simulink model "sim_complete"  (R2015a)
settings: Solver=ode45  StartTime=0.0  StopTime=10.0  RelTol=1e-3
values from neighbouring files (symbols this model uses):
  params = catstruct(params, sys.params_str)    [double_lqg.m]    (also in load_mechanism_params.m = params(1:13); load_params.m = [g, m0, b0,                m1, I1, b1, L1, L1_cg,           ; load_single_mechanism_params.m = params(1:8); load_single_params.m = [g, m0, b0,                m1, I1, b1, L1, L1_cg,           )
libraries: aerolibutil x1
settings Model: Creator=BPeixoto  LastModifiedBy=BPeixoto

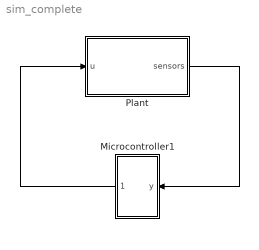
== system sim_complete ==
  Microcontroller1 : Subsystem
  Plant : Subsystem
  wires:
  Microcontroller1/1(PWM) -> Plant/1(u)
  Plant/1(sensors) -> Microcontroller1/1(y)

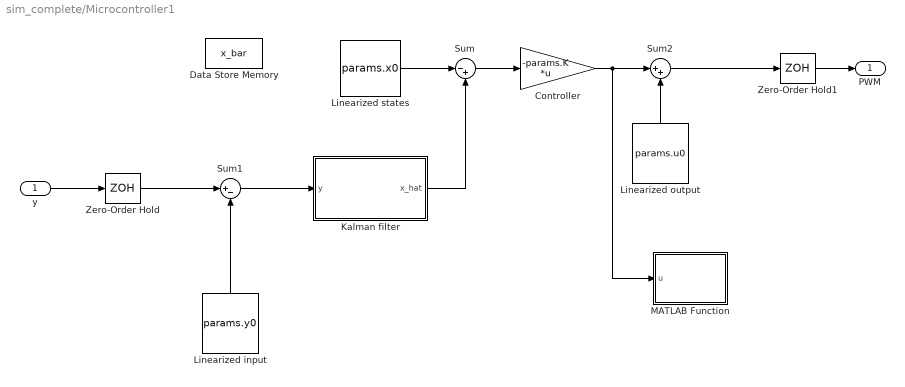
== system sim_complete/Microcontroller1 ==
  y : Inport
  Controller : Gain  Gain=-params.K  Multiplication=Matrix(K*u)
  Data Store Memory : DataStoreMemory  DataStoreName=x_bar  ReadBeforeWriteMsg=warning  WriteAfterWriteMsg=warning  WriteAfterReadMsg=warning  InitialValue=zeros(6, 1)  OutDataTypeStr=double
  Kalman filter : MATLAB Function  TreatAsAtomicUnit=on
  Linearized input : Constant  Value=params.y0
  Linearized output : Constant  Value=params.u0
  Linearized states : Constant  Value=params.x0
  MATLAB Function : MATLAB Function  TreatAsAtomicUnit=on
  Sum : Sum  Inputs=|-+
  Sum1 : Sum  Inputs=|+-
  Sum2 : Sum  Inputs=|++
  Zero-Order Hold : ZeroOrderHold  SampleTime=params.ts
  Zero-Order Hold1 : ZeroOrderHold  SampleTime=params.ts
  PWM : Outport
  wires:
  y/1 -> Zero-Order Hold/1
  Linearized states/1 -> Sum/1
  Sum/1 -> Controller/1
  Linearized input/1 -> Sum1/2
  Zero-Order Hold/1 -> Sum1/1
  Controller/1 -> MATLAB Function/1(u), Sum2/1
  Linearized output/1 -> Sum2/2
  Sum1/1 -> Kalman filter/1(y)
  Sum2/1 -> Zero-Order Hold1/1
  Zero-Order Hold1/1 -> PWM/1
  Kalman filter/1(x_hat) -> Sum/2

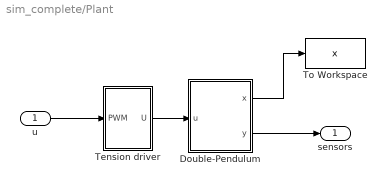
== system sim_complete/Plant ==
  u : Inport
  Double-Pendulum : Subsystem
  Tension driver : Subsystem
  To Workspace : ToWorkspace  VariableName=x  SaveFormat=Timeseries  SampleTime=-1
  sensors : Outport
  wires:
  Double-Pendulum/2(y) -> sensors/1
  Double-Pendulum/1(x) -> To Workspace/1
  u/1 -> Tension driver/1(PWM)
  Tension driver/1(U) -> Double-Pendulum/1(u)

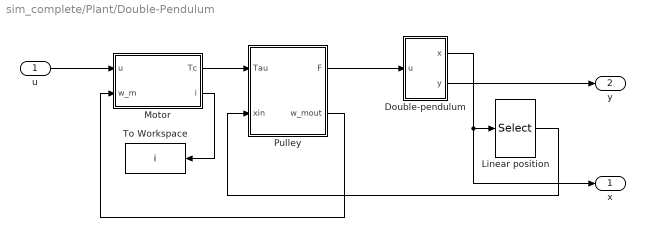
== system sim_complete/Plant/Double-Pendulum ==
  u : Inport
  Double-pendulum : Subsystem
  Linear position : Selector  InputPortWidth=6  Indices=[1]
  Motor : MATLAB Function  TreatAsAtomicUnit=on
  Pulley : Subsystem
  To Workspace : ToWorkspace  VariableName=i  SaveFormat=Timeseries  SampleTime=-1
  x : Outport
  y : Outport  Port=2
  wires:
  u/1 -> Motor/1(u)
  Double-pendulum/1(x) -> x/1, Linear position/1
  Motor/2(i) -> To Workspace/1
  Double-pendulum/2(y) -> y/1
  Motor/1(Tc) -> Pulley/1(Tau)
  Linear position/1 -> Pulley/2(xin)
  Pulley/2(w_mout) -> Motor/2(w_m)
  Pulley/1(F) -> Double-pendulum/1(u)

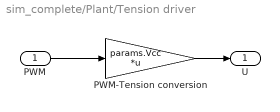
== system sim_complete/Plant/Tension driver ==
  PWM : Inport
  PWM-Tension conversion : Gain  Gain=params.Vcc  Multiplication=Matrix(K*u)
  U : Outport
  wires:
  PWM/1 -> PWM-Tension conversion/1
  PWM-Tension conversion/1 -> U/1

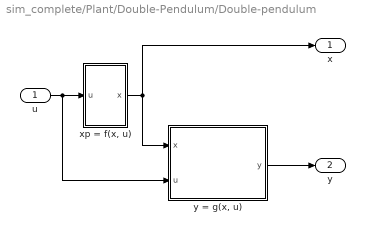
== system sim_complete/Plant/Double-Pendulum/Double-pendulum ==
  u : Inport
  "xp = f(x, u)" : Subsystem
  "y = g(x, u)" : MATLAB Function  TreatAsAtomicUnit=on
  x : Outport
  y : Outport  Port=2
  wires:
  u/1 -> "y = g(x, u)"/2(u), "xp = f(x, u)"/1(u)
  "y = g(x, u)"/1(y) -> y/1
  "xp = f(x, u)"/1(x) -> x/1, "y = g(x, u)"/1(x)

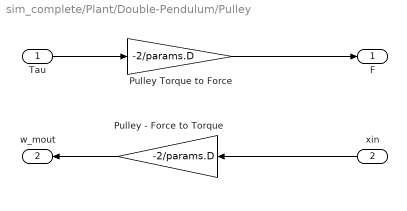
== system sim_complete/Plant/Double-Pendulum/Pulley ==
  Tau : Inport
  xin : Inport  Port=2
  Pulley Torque to Force : Gain  Gain=-2/params.D
  Pulley - Force to Torque : Gain  Gain=-2/params.D
  F : Outport
  w_mout : Outport  Port=2
  wires:
  Pulley Torque to Force/1 -> F/1
  Tau/1 -> Pulley Torque to Force/1
  xin/1 -> Pulley - Force to Torque/1
  Pulley - Force to Torque/1 -> w_mout/1

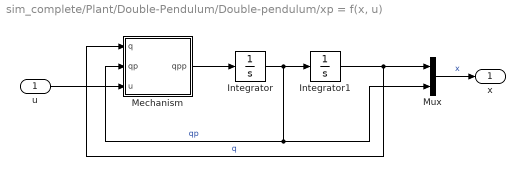
== system sim_complete/Plant/Double-Pendulum/Double-pendulum/xp = f(x, u) ==
  u : Inport
  Integrator : Integrator  InitialCondition=params.qp0
  Integrator1 : Integrator  InitialCondition=params.q0
  Mechanism : Subsystem
  Mux : Mux  Inputs=2
  x : Outport
  wires:
  Mux/1 -> x/1  "x"
  u/1 -> Mechanism/3(u)
  Integrator/1 -> Integrator1/1, Mechanism/2(qp), Mux/2  "qp"
  Mechanism/1(qpp) -> Integrator/1
  Integrator1/1 -> Mux/1, Mechanism/1(q)  "q"

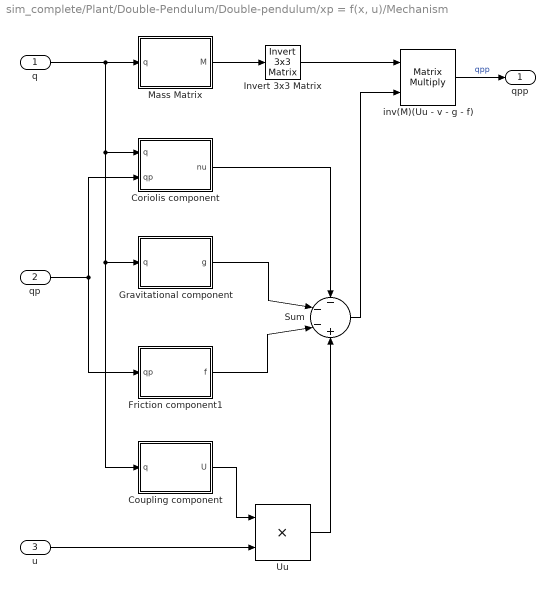
== system sim_complete/Plant/Double-Pendulum/Double-pendulum/xp = f(x, u)/Mechanism ==
  q : Inport
  qp : Inport  Port=2
  u : Inport  Port=3
  Coriolis component : MATLAB Function  TreatAsAtomicUnit=on
  Coupling component : MATLAB Function  TreatAsAtomicUnit=on
  Friction component1 : MATLAB Function  TreatAsAtomicUnit=on
  Gravitational component : MATLAB Function  TreatAsAtomicUnit=on
  Invert 3x3 Matrix : aerolibutil/Invert  3x3 Matrix
  Mass Matrix : MATLAB Function  TreatAsAtomicUnit=on
  Sum : Sum  Inputs=-|-|-|+
  Uu : Product  RndMeth=Nearest
  inv(M)(Uu - v - g - f) : Product  Multiplication=Matrix(*)  OutDataTypeStr=Inherit: Inherit via back propagation  SaturateOnIntegerOverflow=on  InputSameDT=on
  qpp : Outport
  wires:
  Mass Matrix/1(M) -> Invert 3x3 Matrix/1
  Coriolis component/1(nu) -> Sum/1
  qp/1 -> Coriolis component/2(qp), Friction component1/1(qp)
  q/1 -> Coupling component/1(q), Gravitational component/1(q), Coriolis component/1(q), Mass Matrix/1(q)
  Gravitational component/1(g) -> Sum/2
  Friction component1/1(f) -> Sum/3
  Invert 3x3 Matrix/1 -> inv(M)(Uu - v - g - f)/1
  Sum/1 -> inv(M)(Uu - v - g - f)/2
  inv(M)(Uu - v - g - f)/1 -> qpp/1  "qpp"
  Coupling component/1(U) -> Uu/1
  u/1 -> Uu/2
  Uu/1 -> Sum/4

== matlab function sim_complete/Plant/Double-Pendulum/Double-pendulum/xp = f(x, u)/Mechanism/Coriolis component ==
  settings: updateMethod=DISCRETE  sampleTime=params.ts
  data: q input; qp input; nu output; params parameter
function nu = corvec(q, qp, params)
    % Coriolis 'vector
    nu = zeros(3, 1);
    
    % Coupled mass matrix
    nu(1) = -params.m2*params.L2_cg*sin(q(2) + q(3))*(qp(2) + qp(3)^2 ...
            -(params.m2*params.L1 + params.m1*params.L1_cg)*sin(q(2))*qp(3)^2);
    nu(2) = -params.m2*qp(3)*(2*qp(2) + qp(3))*params.L2_cg*params.L1*sin(q(3));
    nu(3) = params.m2*(qp(2)^2)*params.L2_cg*params.L1*sin(q(3));
end

== matlab function sim_complete/Plant/Double-Pendulum/Double-pendulum/xp = f(x, u)/Mechanism/Coupling component ==
  settings: updateMethod=DISCRETE  sampleTime=params.ts
  data: q input; U output
function U = Uvec(q)
    U = [1; 0; 0];
end

== matlab function sim_complete/Microcontroller1/Kalman filter ==
  data: y input; params parameter; u_ant data_store_memory; x_hat_ant data_store_memory; x_hat output
function x_hat = kalman_filter(y, params)
    % First assignemnt
    global x_bar;
    
    % Main matrices
    L = params.L;
    Phi = params.Phi;
    Gamma = params.Gamma;
    C = params.C;
    
    % Time and measurement update
    x_hat = x_bar + L*(y - C*x_bar);
    x_bar = Phi*x_hat + Gamma*u_ant;
end

== matlab function sim_complete/Microcontroller1/MATLAB Function ==
  data: u input; u_ant data_store_memory
function save_uant(u)    
    global u_ant;    
    u_ant = u;
end

== matlab function sim_complete/Plant/Double-Pendulum/Motor ==
  settings: updateMethod=DISCRETE  sampleTime=params.ts
  data: Tc output; i output; u input; w_m input; params parameter
function [Tc, i] = motor(u, w_m, params)
    % Motor parameters
    % Simplifications: 
    %   Negligible pulley inertia and stator inductance
    Ra = params.Ra;
    Kt = params.Kt;
    Ke = params.Ke;
    
    % Exerted Torque
    Tc = (Kt/Ra)*(u - Ke*w_m);
    i = Tc/Kt;

== matlab function sim_complete/Plant/Double-Pendulum/Double-pendulum/xp = f(x, u)/Mechanism/Friction component1 ==
  settings: updateMethod=DISCRETE  sampleTime=params.ts
  data: qp input; f output; params parameter
function f = fvec(qp, params)
    % Friction vector
    f = zeros(3, 1);
    
    % Coupled mass matrix
    f(1) = params.b0*qp(1);
    f(2) = params.b1*qp(2);
    f(3) = params.b2*qp(3);
end

== matlab function sim_complete/Plant/Double-Pendulum/Double-pendulum/xp = f(x, u)/Mechanism/Gravitational component ==
  settings: updateMethod=DISCRETE  sampleTime=params.ts
  data: q input; g output; params parameter
function g = gvec(q, params)
    % Gravitational component
    g = zeros(3, 1);
    
    % Coupled mass matrix
    g(1) = 0;
    g(2) = params.m2*params.g*(params.L1*sin(q(2)) + ...
           params.L2_cg*sin(q(2) + q(3))) + ...
           params.m1*params.L1_cg*params.g*sin(q(2));
    g(3) = params.m2*params.g*params.L2_cg*sin(q(2) + q(3));
end

== matlab function sim_complete/Plant/Double-Pendulum/Double-pendulum/xp = f(x, u)/Mechanism/Mass Matrix ==
  settings: updateMethod=DISCRETE  sampleTime=params.ts
  data: q input; M output; params parameter
function M = mmatrix(q, params)
    % Mass matrix
    M = zeros(3, 3);
    
    % Coupled mass matrix
    M(1,1) = params.m0 + params.m1 + params.m2;
    
    M(2,2) = params.m2*params.L1^2 + params.m1*params.L1_cg^2 +...
             params.m2*params.L2_cg^2 + ...
             params.I1 + params.I2 + 2*params.m2*params.L1*params.L2_cg*cos(q(3));
    
    M(3,3) = params.m2*params.L2_cg^2 + params.I2;
         
    M(1,2) = params.m2*params.L2_cg*cos(q(2) + q(3)) + ...
            (params.m2*params.L1 + params.m1*params.L1_cg)*cos(q(2));
    
    M(1,3) = params.m2*params.L2_cg*cos(q(2) + q(3));
    
    M(2,3) = params.m2*params.L2_cg^2 + params.I2 + ...
             params.m2*params.L1*params.L2_cg*cos(q(3));
    
    M(2,1) = M(1,2);
    M(3,1) = M(1,3);
    M(3,2) = M(2,3);
end

== matlab function sim_complete/Plant/Double-Pendulum/Double-pendulum/y = g(x, u) ==
  settings: updateMethod=DISCRETE  sampleTime=params.ts
  data: x input; y output; u input
function y = system_output(x, u)
    y = [x(1); x(2); x(3)];
end
